simulink model "dc_motor"  (R2023b)
settings: Solver=FixedStepAuto  StartTime=0.0  StopTime=inf  FixedStep=0.02  RelTol=1e-3  EnableMultiTasking=on
libraries: arduinolib x4
settings Model: ExtModeTrigDuration=2  Creator=konsta  LastModifiedBy=konsta
settings OptimizationCC: EnhancedBackFolding=on  PassReuseOutputArgsAs=Individual arguments  ZeroExternalMemoryAtStartup=off  ZeroInternalMemoryAtStartup=off  MaxStackSize=64  OptimizeBlockOrder=speed  DifferentSizesBufferReuse=on  OptimizationCustomize=off  EfficientTunableParamExpr=on
settings DebuggingCC: ParameterTunabilityLossMsg=error
settings HardwareCC: ProdBitPerInt=16  ProdBitPerPointer=16  ProdBitPerSizeT=16  ProdBitPerPtrDiffT=16  ProdLargestAtomicFloat=None  ProdWordSize=8  ProdHWDeviceType=Atmel->AVR  UseEmbeddedCoderFeatures=off  UseSimulinkCoderFeatures=off
settings SFSimCC: MATLABDynamicMemAlloc=off
settings RTWCC: Description=Embedded Coder  SystemTargetFile=ert.tlc  HardwareBoard=Arduino Uno  TemplateMakefile=ert_default_tmf  Toolchain=Arduino AVR  BuildConfiguration=Faster Runs
settings CodeAppCC: ForceParamTrailComments=on  IgnoreCustomStorageClasses=off  OperatorAnnotations=on  SimulinkDataObjDesc=on  SFDataObjDesc=on  InsertBlockDesc=on
settings ERTTargetCC: SupportContinuousTime=on  SupportNonInlinedSFcns=on  SupportVariableSizeSignals=on  ExtModeTransport=3  ExtModeStaticAlloc=on  ExtModeAutomaticAllocSize=off  ExtModeStaticAllocSize=250  ExtModeMexFile=ext_xcp  ExtModeIntrfLevel=Level2 - Open

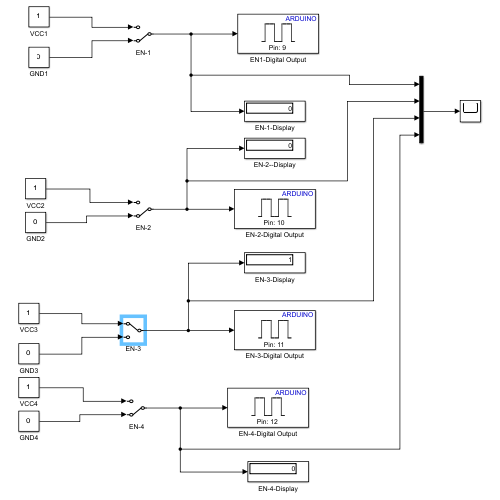
[thumbnail: Simulink's stored preview of the top-level diagram]
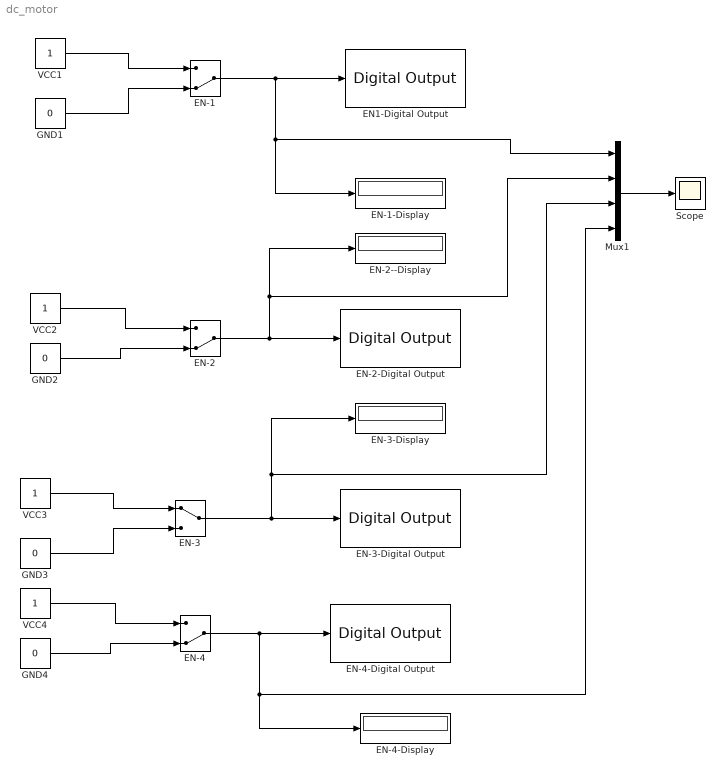
== system dc_motor ==
  EN-1 : ManualSwitch  CurrentSetting=0
  EN-1-Display : Display
  EN-2 : ManualSwitch  CurrentSetting=0
  EN-2--Display : Display
  EN-2-Digital Output : arduinolib/Digital Output  pinNumber=10  Direction=output  blockPlatform=arduino
  EN-3 : ManualSwitch
  EN-3-Digital Output : arduinolib/Digital Output  pinNumber=11  Direction=output  blockPlatform=arduino
  EN-3-Display : Display
  EN-4 : ManualSwitch  CurrentSetting=0
  EN-4-Digital Output : arduinolib/Digital Output  pinNumber=12  Direction=output  blockPlatform=arduino
  EN-4-Display : Display
  EN1-Digital Output : arduinolib/Digital Output  pinNumber=9  Direction=output  blockPlatform=arduino
  GND{1..4} (4 alike) : Constant  Value=0
  Mux1 : Mux
  Scope : Scope
  VCC{1..4} (4 alike) : Constant
  wires:
  VCC1/1 -> EN-1/1
  GND1/1 -> EN-1/2
  EN-1/1 -> Mux1/1, EN-1-Display/1, EN1-Digital Output/1
  VCC2/1 -> EN-2/1
  GND2/1 -> EN-2/2
  EN-2/1 -> Mux1/2, EN-2--Display/1, EN-2-Digital Output/1
  Mux1/1 -> Scope/1
  VCC3/1 -> EN-3/1
  EN-4/1 -> EN-4-Display/1, Mux1/4, EN-4-Digital Output/1
  GND4/1 -> EN-4/2
  VCC4/1 -> EN-4/1
  GND3/1 -> EN-3/2
  EN-3/1 -> Mux1/3, EN-3-Display/1, EN-3-Digital Output/1
